simulink model "lab3_07_pi_tuned"  (R2025b)
settings: Solver=ode45  StartTime=0.0  StopTime=30.0  MaxStep=0.01  RelTol=1e-6
settings Model: Creator=Boris  LastModifiedBy=Boris

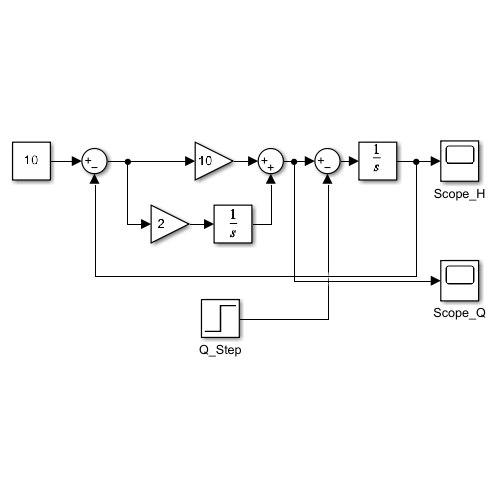
[thumbnail: Simulink's stored preview of the top-level diagram]
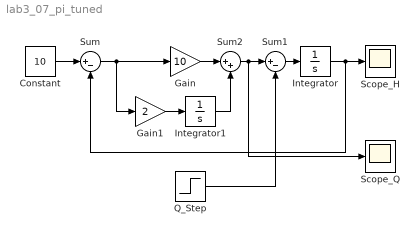
== system lab3_07_pi_tuned ==
  Constant : Constant  Value=10
  Gain : Gain  Gain=10
  Gain1 : Gain  Gain=2
  Integrator : Integrator
  Integrator1 : Integrator
  Q_Step : Step  Time=6  After=2  SampleTime=0
  Scope_H : Scope
      settings: ActiveDisplayYMinimum=-12.737485297214677  ActiveDisplayYMaximum=18.6045938448039
  Scope_Q : Scope
      settings: ActiveDisplayYMinimum=-13.733789799742423  ActiveDisplayYMaximum=19.175393299377088
  Sum : Sum  Inputs=|+-
  Sum1 : Sum  Inputs=|+-
  Sum2 : Sum  Inputs=|++
  wires:
  Integrator/1 -> Sum/2, Scope_H/1
  Constant/1 -> Sum/1
  Sum/1 -> Gain1/1, Gain/1
  Gain1/1 -> Integrator1/1
  Sum1/1 -> Integrator/1
  Gain/1 -> Sum2/1
  Sum2/1 -> Scope_Q/1, Sum1/1
  Integrator1/1 -> Sum2/2
  Q_Step/1 -> Sum1/2
